simulink library "ESTS_VVSO_WHL_LatLoadTransf"  (R2024b)
settings: Solver=VariableStepAuto  StartTime=0.0  StopTime=10.0  RelTol=1e-3
undefined symbols (not defined in the file): c_GravConst_mps2
settings Model: Creator=blatak  LastModifiedBy=blatak
settings ModelReferenceCC: EnableRefExpFcnMdlSchedulingChecks=on
settings RTWCC: GPUComputeCapability=3.5

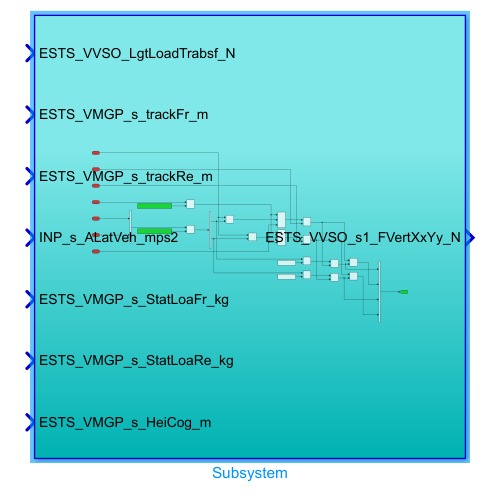
[thumbnail: Simulink's stored preview of the top-level diagram]
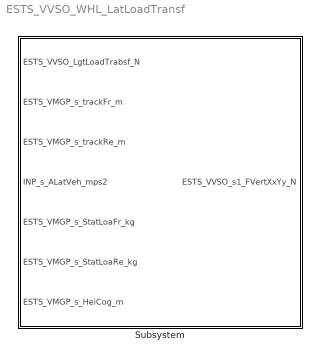
== system ESTS_VVSO_WHL_LatLoadTransf ==
  Subsystem : Subsystem

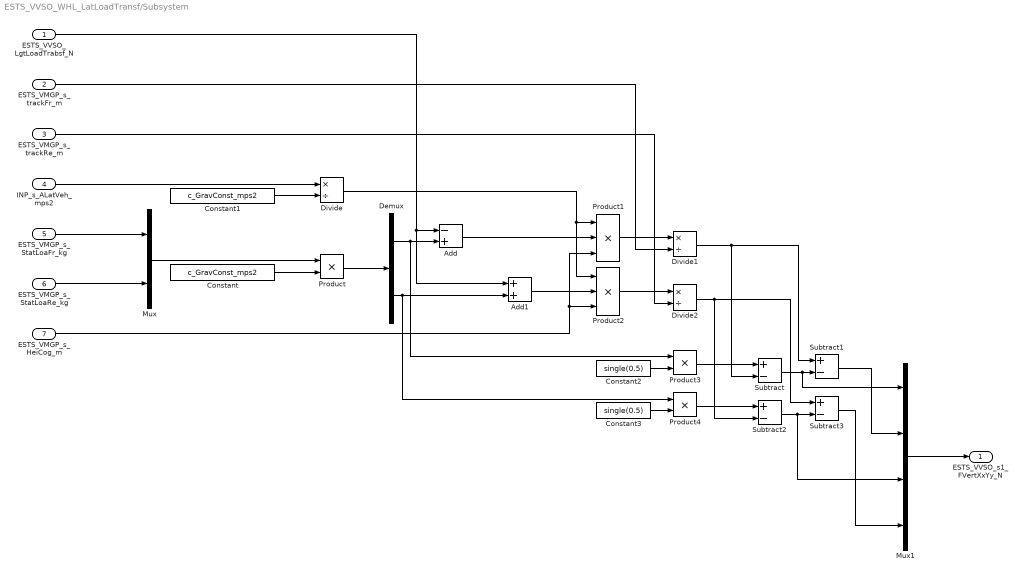
== system ESTS_VVSO_WHL_LatLoadTransf/Subsystem ==
  ESTS_VVSO_LgtLoadTrabsf_N : Inport
  ESTS_VMGP_s_trackFr_m : Inport  Port=2
  ESTS_VMGP_s_trackRe_m : Inport  Port=3
  INP_s_ALatVeh_mps2 : Inport  Port=4
  ESTS_VMGP_s_StatLoaFr_kg : Inport  Port=5
  ESTS_VMGP_s_StatLoaRe_kg : Inport  Port=6
  ESTS_VMGP_s_HeiCog_m : Inport  Port=7
  Add : Sum  Inputs=-+
  Add1 : Sum
  Constant : Constant  Value=c_GravConst_mps2
  Constant1 : Constant  Value=c_GravConst_mps2
  Constant2 : Constant  Value=single(0.5)
  Constant3 : Constant  Value=single(0.5)
  Demux : Demux  Outputs=2
  Divide : Product  Inputs=*/  RndMeth=Zero  SaturateOnIntegerOverflow=on
  Divide1 : Product  Inputs=*/  RndMeth=Zero  SaturateOnIntegerOverflow=on
  Divide2 : Product  Inputs=*/  RndMeth=Zero  SaturateOnIntegerOverflow=on
  Mux : Mux  Inputs=2
  Mux1 : Mux
  Product : Product
  Product1 : Product  Inputs=3
  Product2 : Product  Inputs=3
  Product3 : Product
  Product4 : Product
  Subtract{,1..3} (4 alike) : Sum  Inputs=+-
  ESTS_VVSO_s1_FVertXxYy_N : Outport
  wires:
  ESTS_VMGP_s_StatLoaRe_kg/1 -> Mux/2
  ESTS_VMGP_s_StatLoaFr_kg/1 -> Mux/1
  Mux/1 -> Product/1
  Constant/1 -> Product/2
  Product/1 -> Demux/1
  Demux/1 -> Product3/1, Add/2
  ESTS_VVSO_LgtLoadTrabsf_N/1 -> Add/1, Add1/1
  Demux/2 -> Product4/1, Add1/2
  Add/1 -> Product1/2
  Add1/1 -> Product2/2
  INP_s_ALatVeh_mps2/1 -> Divide/1
  Constant1/1 -> Divide/2
  ESTS_VMGP_s_HeiCog_m/1 -> Product1/3, Product2/3
  Divide/1 -> Product2/1, Product1/1
  Product1/1 -> Divide1/1
  Product2/1 -> Divide2/1
  ESTS_VMGP_s_trackFr_m/1 -> Divide1/2
  ESTS_VMGP_s_trackRe_m/1 -> Divide2/2
  Constant2/1 -> Product3/2
  Constant3/1 -> Product4/2
  Product3/1 -> Subtract/1
  Subtract/1 -> Mux1/1, Subtract1/2
  Divide1/1 -> Subtract/2, Subtract1/1
  Product4/1 -> Subtract2/1
  Divide2/1 -> Subtract3/1, Subtract2/2
  Subtract2/1 -> Mux1/3, Subtract3/2
  Subtract1/1 -> Mux1/2
  Subtract3/1 -> Mux1/4
  Mux1/1 -> ESTS_VVSO_s1_FVertXxYy_N/1
